simulink model "PIDControl"  (R2018a)
settings: Solver=ode45  StartTime=0.0  StopTime=50  RelTol=1e-3  EnableMultiTasking=on
values from neighbouring files (symbols this model uses):
  gain = [kx;kx_d;kx_i;        ky;ky_d;ky_i;        kz;kz_d;kz_i;        k_phi;kphi_d;kphi_i;        k_theta;ktheta_d;ktheta_i;        k_psi;kpsi_d;kpsi_i]    [InitQuadModel4Simulink.m]
  initialCondition = [x0 vx0 y0 vy0 z0 vz0 phi0 p0 theta0 q0 psi0 r0]'    [InitQuadModel4Simulink.m]
  par = [m;m1;Ix;Iy;Iz;Ir;Om_r;d;l;g]    [InitQuadModel4Simulink.m]
  regval = [x_d;y_d;z_d;phi_d;theta_d;psi_d]    [InitQuadModel4Simulink.m]
settings Model: Creator=marilena  LastModifiedBy=Marilena
settings DataIOCC: LimitDataPoints=on  SaveFormat=Array  SignalLoggingSaveFormat=ModelDataLogs
settings OptimizationCC: ExpressionDepthLimit=2147483647  LifeSpan=inf
settings DebuggingCC: UnderspecifiedInitializationDetection=Classic  MergeDetectMultiDrivingBlocksExec=none  SolverPrmCheckMsg=warning  FcnCallInpInsideContextMsg=warning  StateNameClashWarn=warning  SFUnexpectedBacktrackingDiag=warning  SFNoUnconditionalDefaultTransitionDiag=warning  SFExecutionAtInitializationDiag=none
settings HardwareCC: ProdBitPerPointer=32  ProdBitPerSizeT=32  ProdBitPerPtrDiffT=32  ProdLargestAtomicFloat=None  ProdIntDivRoundTo=Undefined  ProdEndianess=Unspecified  ProdWordSize=32  ProdHWDeviceType=32-bit Generic
settings ModelReferenceCC: PropagateSignalLabelsOutOfModel=off
settings CodeAppCC: StateflowObjectComments=on
settings GRTTargetCC: TargetLangStandard=C89/C90 (ANSI)  GeneratePreprocessorConditionals=Disable all
settings ConfigComp: CovMetricSettings=dw  CovHtmlReporting=on  CovSaveCumulativeToWorkspaceVar=on  CovSaveSingleToWorkspaceVar=on  CovExternalEMLEnable=off  CovSFcnEnable=off

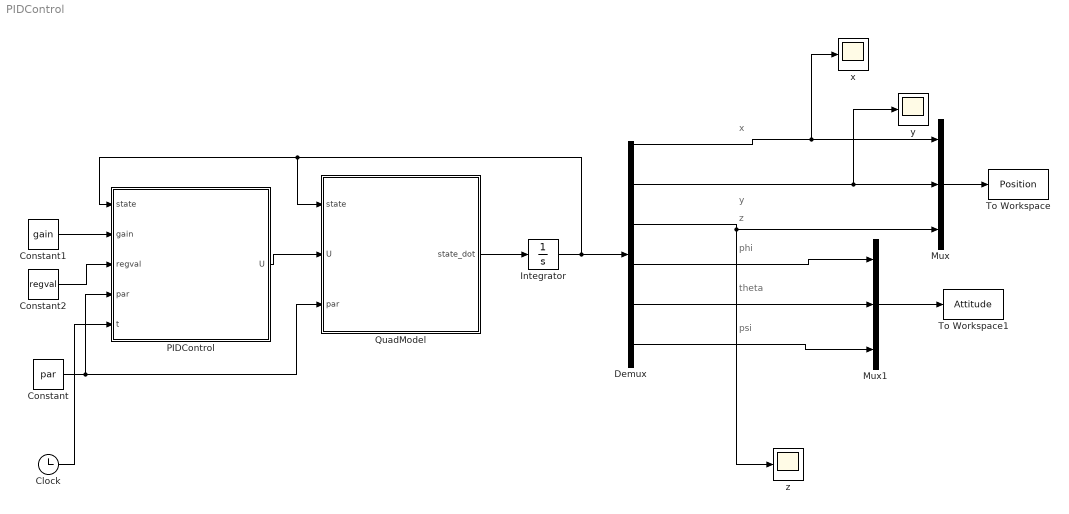
== system PIDControl ==
  note: x
  note: y
  note: z
  note: phi
  note: theta
  note: psi
  Clock : Clock
  Constant : Constant  Value=par
  Constant1 : Constant  Value=gain
  Constant2 : Constant  Value=regval
  Demux : Demux  Outputs=12
  Integrator : Integrator  InitialCondition=initialCondition
  Mux : Mux  Inputs=3
  Mux1 : Mux  Inputs=3
  "PIDControl " : MATLAB Function  TreatAsAtomicUnit=on
  QuadModel : MATLAB Function  TreatAsAtomicUnit=on
  To Workspace : ToWorkspace  VariableName=Position  SaveFormat=Structure With Time  SampleTime=-1
  To Workspace1 : ToWorkspace  VariableName=Attitude  SaveFormat=Structure With Time  SampleTime=-1
  x : Scope
  "y " : Scope
  z : Scope
  wires:
  Demux/1 -> x/1, Mux/1
  Demux/3 -> "y "/1, Mux/2
  Demux/5 -> z/1, Mux/3
  Demux/7 -> Mux1/1
  Demux/11 -> Mux1/3
  QuadModel/1(state_dot) -> Integrator/1
  "PIDControl "/1(U) -> QuadModel/2(U)
  Constant2/1 -> "PIDControl "/3(regval)
  Constant1/1 -> "PIDControl "/2(gain)
  Integrator/1 -> QuadModel/1(state), "PIDControl "/1(state), Demux/1
  Constant/1 -> QuadModel/3(par), "PIDControl "/4(par)
  Demux/9 -> Mux1/2
  Mux/1 -> To Workspace/1
  Mux1/1 -> To Workspace1/1
  Clock/1 -> "PIDControl "/5(t)

== matlab function PIDControl/PIDControl  ==
  data: state input; U output; gain input; regval input; par input; t input
function U = PID_C(state,gain,regval,par,t)

%model parameters
m=par(1);
m1=par(2);
Ix=par(3);
Iy=par(4);
Iz=par(5);
Ir=par(6);
Om_r=par(7);
d=par(8);
l=par(9);
g=par(10);

%controller gains
kx=gain(1);
kx_d=gain(2);
kx_i=gain(3);

ky=gain(4);
ky_d=gain(5);
ky_i=gain(6);

kz=gain(7);
kz_d=gain(8);
kz_i=gain(9);

k_phi=gain(10);
kphi_d=gain(11);
kphi_i=gain(12);

k_theta=gain(13);
ktheta_d=gain(14);
ktheta_i=gain(15);

k_psi=gain(16);
kpsi_d=gain(17);
kpsi_i=gain(18);

%%%% reference signals %%%%%%

% %regulation values
% x_d=regval(1);
% y_d=regval(2);
% z_d=regval(3);
% psi_d=regval(6);
% vx_d = 0;
% vy_d = 0;
% vz_d = 0;
% vxdot_d = 0;
% vydot_d = 0;
% vzdot_d = 0;

%desired trajectories 
%spirale
psi_d=regval(6);

x_d = cos(t);
y_d = sin(t);
z_d = 2*t;
vx_d = -sin(t);
vy_d = cos(t);
vz_d = 2;
vxdot_d = -cos(t);
vydot_d = -sin(t);
vzdot_d = 0;
%%%%  %%%%%%


%position
x=state(1);
vx=state(2);
y=state(3);
vy=state(4);
z=state(5);
vz=state(6);

%attitude
phi=state(7);
dphi=state(8);
theta=state(9);
dtheta=state(10);
psi=state(11);
dpsi=state(12);

% height control
stab_z=(g + kz*(z_d -z) + kz_d*(vz_d-vz));
fl_z=(m/(cos(phi)*cos(theta)));
T=fl_z*stab_z;

%desired thrust direction
Tx=(m/T)*(kx*(x_d-x)+kx_d*(vx_d-vx)+vxdot_d);
Ty=(m/T)*(ky*(y_d-y)+ky_d*(vy_d-vy)+vydot_d);

%desired attitude from desired thrust direction
phi_d=asin(Tx*sin(psi)-Ty*cos(psi));
theta_d=asin((Tx*cos(psi)+Ty*sin(psi))/cos(phi_d));

tau_phi=Ix*(k_phi * (phi_d - phi) + kphi_d * (-dphi));
tau_theta=Iy*(k_theta * (theta_d - theta) + ktheta_d * (-dtheta));
tau_psi=Iz*(k_psi * (psi_d - psi) + kpsi_d * (-dpsi));

U = [T, tau_phi, tau_theta, tau_psi]';

== matlab function PIDControl/QuadModel ==
  data: state input; U input; state_dot output; par input
function state_dot = quadrotor_model(state,U,par)

%model parameters
m=par(1);
m1=par(2);
Ix=par(3);
Iy=par(4);
Iz=par(5);
Ir=par(6);
Om_r=par(7);
d=par(8);
l=par(9);
g=par(10);

%position
x=state(1);
vx=state(2);
y=state(3);
vy=state(4);
z=state(5);
vz=state(6);

%attitude
phi=state(7);
dphi=state(8);
theta=state(9);
dtheta=state(10);
psi=state(11);
dpsi=state(12);

%control
T=U(1);
tau_phi=U(2);
tau_theta=U(3);
tau_psi=U(4);

%dynamics

%NOTE: to obtain a model in the  
%NED(=North-East-Down) frame 
%put a minus sign before the rhs of the vxdot, vydot, vzdot equations 
% and modify accordingly 
%also the control equations from the slides...


xdot=vx;
vxdot = (T/m)*(cos(phi)*sin(theta)*cos(psi)+sin(phi)*sin(psi));

ydot=vy;
vydot = (T/m)*(cos(phi)*sin(theta)*sin(psi)-sin(phi)*cos(psi));

zdot=vz;
vzdot = (- g + (T/m)*(cos(phi)*cos(theta)));

phidot=dphi;
dphidot =  ((Iy-Iz)/Ix)*dtheta*dpsi + (Ir/Ix)*dtheta*Om_r +(l/Ix)*tau_phi; %;

thetadot=dtheta;
dthetadot = ((Iz-Ix)/Iy)*dphi*dpsi - (Ir/Iy)*dphi*Om_r +(l/Iy)*tau_theta;  %;

psidot=dpsi;
dpsidot =  ((Ix-Iy)/Iz)*dphi*dtheta + (1/Iz)*tau_psi; %;

state_dot = [xdot, vxdot, ydot, vydot, zdot, vzdot, phidot, dphidot, thetadot, dthetadot, psidot, dpsidot]';
